simulink model "k1visex"  (Simulink 8.5)
settings: Solver=ode45  StartTime=0.0  StopTime=10.0  RelTol=1e-3
libraries: cdsFilt x6, cdsIPCx x4, cdsEpicsOut x2, cdsAdcx0 x1, dac x1, TYPEC_MASTER x1, cdsParameters x1
settings Model: Creator=controls  LastModifiedBy=controls
settings DataIOCC: SignalLoggingSaveFormat=Dataset
settings OptimizationCC: ExpressionDepthLimit=128
settings DebuggingCC: UnderspecifiedInitializationDetection=Simplified  MergeDetectMultiDrivingBlocksExec=error  FcnCallInpInsideContextMsg=EnableAllAsError  StateNameClashWarn=none
settings GRTTargetCC: CombineOutputUpdateFcns=on  GRTInterface=off

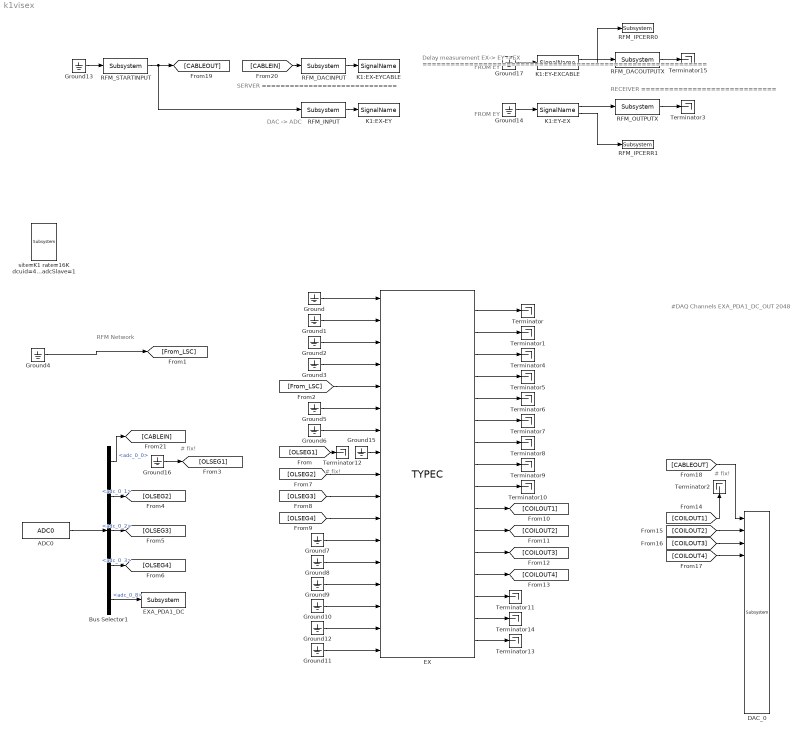
== system k1visex ==
  note: RFM Network
  note: #DAQ Channels
      |
      | EXA_PDA1_DC_OUT 2048
  note: FROM EY
  note: DAC -> ADC
  note: FROM EY
  note: Delay measurement
      | EX-> EY ->EX
      | =============================================================
  note: SERVER
      | =============================
  note: RECEIVER
      | =============================
  note: # fix!
  note: # fix!
  note: # fix!
  ADC0 : cdsAdcx0/ADC0  Tag=cdsAdc  Description=|
      | type-GSC_16AI64SSA
      | card_num=0
      settings: AttributesFormatString=%<Description>\n%<Tag>
  Bus Selector1 : BusSelector  Description=ADC Selector  OutputSignals=adc_0_0,adc_0_1,adc_0_2,adc_0_3,adc_0_8
      settings: AttributesFormatString=%<Description>
  DAC_0 : dac/Subsystem  Description=|
      | type=GSC_16AO16,
      | card_num=0
      settings: AttributesFormatString=%<Description>
  EX : TYPEC_MASTER/TYPEC  Description=TYPEC MASTER
      settings: AttributesFormatString=%<Description>
  EXA_PDA1_DC : cdsFilt/Subsystem  Tag=cdsFilt  Description=|
      | Purpose:                                                                                                                                                                                                                                  
      | Standard CDS IIR filter module.                                                                                                                                                                                                           
      |                                                                                                                                                                                                                                           
      | Operation:                                                                                                                                                                                                                                
      | Consists of 10 second order section IIR filters, plus a ramped gain stage. In FE code, also provides pre-defined test points and excitation channel inputs. The filter coefficients are defined in the LIGO system using the 'foton' tool.
      |                                                                                                                                                                                                                                           
      | Usage:                                                                                                                                                                                                                                    
      | Name the part with the desired filter module name.
      settings: AttributesFormatString=%<Tag>
  Ground{,1..17} (18 alike) : Ground
  K1:EX-EY : cdsIPCx/SignalName  Tag=cdsIPCx_RFM  Description=card=0
      settings: AttributesFormatString=%<Description>\n%<Tag>
  K1:EX-EYCABLE : cdsIPCx/SignalName  Tag=cdsIPCx_RFM  Description=card=0
      settings: AttributesFormatString=%<Description>\n%<Tag>
  K1:EY-EX : cdsIPCx/SignalName  Tag=cdsIPCx_RFM  Description=card=0
      settings: AttributesFormatString=%<Description>\n%<Tag>
  K1:EY-EXCABLE : cdsIPCx/SignalName  Tag=cdsIPCx_RFM  Description=card=0
      settings: AttributesFormatString=%<Description>\n%<Tag>
  RFM_DACINPUT : cdsFilt/Subsystem  Tag=cdsFilt  Description=|
      | Purpose:                                                                                                                                                                                                                                  
      | Standard CDS IIR filter module.                                                                                                                                                                                                           
      |                                                                                                                                                                                                                                           
      | Operation:                                                                                                                                                                                                                                
      | Consists of 10 second order section IIR filters, plus a ramped gain stage. In FE code, also provides pre-defined test points and excitation channel inputs. The filter coefficients are defined in the LIGO system using the 'foton' tool.
      |                                                                                                                                                                                                                                           
      | Usage:                                                                                                                                                                                                                                    
      | Name the part with the desired filter module name.
      settings: AttributesFormatString=%<Tag>
  RFM_DACOUTPUTX : cdsFilt/Subsystem  Tag=cdsFilt  Description=|
      | Purpose:                                                                                                                                                                                                                                  
      | Standard CDS IIR filter module.                                                                                                                                                                                                           
      |                                                                                                                                                                                                                                           
      | Operation:                                                                                                                                                                                                                                
      | Consists of 10 second order section IIR filters, plus a ramped gain stage. In FE code, also provides pre-defined test points and excitation channel inputs. The filter coefficients are defined in the LIGO system using the 'foton' tool.
      |                                                                                                                                                                                                                                           
      | Usage:                                                                                                                                                                                                                                    
      | Name the part with the desired filter module name.
      settings: AttributesFormatString=%<Tag>
  RFM_INPUT : cdsFilt/Subsystem  Tag=cdsFilt  Description=|
      | Purpose:                                                                                                                                                                                                                                  
      | Standard CDS IIR filter module.                                                                                                                                                                                                           
      |                                                                                                                                                                                                                                           
      | Operation:                                                                                                                                                                                                                                
      | Consists of 10 second order section IIR filters, plus a ramped gain stage. In FE code, also provides pre-defined test points and excitation channel inputs. The filter coefficients are defined in the LIGO system using the 'foton' tool.
      |                                                                                                                                                                                                                                           
      | Usage:                                                                                                                                                                                                                                    
      | Name the part with the desired filter module name.
      settings: AttributesFormatString=%<Tag>
  RFM_IPCERR0 : cdsEpicsOut/Subsystem  Tag=cdsEpicsOutput  Description=|
      | Purpose:                                          
      | Output a FE signal to an EPICS channel.           
      |                                                   
      | Operation:                                        
      | Takes input value and passes it to EPICS record.  
      |                                                   
      | Usage:                                            
      | Name the part with the desired EPICS rrecord name.
      settings: AttributesFormatString=%<Tag>
  RFM_IPCERR1 : cdsEpicsOut/Subsystem  Tag=cdsEpicsOutput  Description=|
      | Purpose:                                          
      | Output a FE signal to an EPICS channel.           
      |                                                   
      | Operation:                                        
      | Takes input value and passes it to EPICS record.  
      |                                                   
      | Usage:                                            
      | Name the part with the desired EPICS rrecord name.
      settings: AttributesFormatString=%<Tag>
  RFM_OUTPUTX : cdsFilt/Subsystem  Tag=cdsFilt  Description=|
      | Purpose:                                                                                                                                                                                                                                  
      | Standard CDS IIR filter module.                                                                                                                                                                                                           
      |                                                                                                                                                                                                                                           
      | Operation:                                                                                                                                                                                                                                
      | Consists of 10 second order section IIR filters, plus a ramped gain stage. In FE code, also provides pre-defined test points and excitation channel inputs. The filter coefficients are defined in the LIGO system using the 'foton' tool.
      |                                                                                                                                                                                                                                           
      | Usage:                                                                                                                                                                                                                                    
      | Name the part with the desired filter module name.
      settings: AttributesFormatString=%<Tag>
  RFM_STARTINPUT : cdsFilt/Subsystem  Tag=cdsFilt  Description=|
      | Purpose:                                                                                                                                                                                                                                  
      | Standard CDS IIR filter module.                                                                                                                                                                                                           
      |                                                                                                                                                                                                                                           
      | Operation:                                                                                                                                                                                                                                
      | Consists of 10 second order section IIR filters, plus a ramped gain stage. In FE code, also provides pre-defined test points and excitation channel inputs. The filter coefficients are defined in the LIGO system using the 'foton' tool.
      |                                                                                                                                                                                                                                           
      | Usage:                                                                                                                                                                                                                                    
      | Name the part with the desired filter module name.
      settings: AttributesFormatString=%<Tag>
  Terminator{,1..15} (16 alike) : Terminator
  site=K1 rate=16K dcuid=42 host=k1ex0 specific_cpu=38 adcSlave=1 : cdsParameters/Subsystem  Tag=cdsParameters  Description=|
      | Purpose:                                                                                                                                                                                                                                
      | Provide system parameters to the FE code generator to properly configure the generated EPICS names, rep rate of the FE controller, and the Data Acquisition node ID for proper storage of data from this FE controller.                 
      |                                                                                                                                                                                                                                         
      | Useage:                                                                                                                                                                                                                                 
      | The part NAME field is used to identify the FE parameters. It must be of the form:                                                                                                                                                      
      | site=                                                                                                                                                                                                                                   
      | rate=                                                                                                                                                                                                                                   
      | dcuid=                                                                                                                                                                                                                                  
      |                                                                                                                                                                                                                                         
      | Where:                                                                                                                                                                                                                                  
      | site= argument may be H1, H2, L1, M1, G1, either as a single argument or multiple, for example site=H1,H2. These are the only names allowed. These will become the first two characters of all EPICS and signal names (for example G1:).
      |                                                                                                                                                                                                                                         
      | rate= may be 2K, 16K, 32K, or 64K                                                                                                                                                                                                       
      |                                                                                                                                                                                                                                         
      | dcuid= is site specific ie it must be unique at each site.
      settings: AttributesFormatString=%<Tag>
  wires:
  ADC0/1 -> Bus Selector1/1
  Ground2/1 -> EX/3
  Ground1/1 -> EX/2
  Ground/1 -> EX/1
  Ground3/1 -> EX/4
  Ground8/1 -> EX/13
  Ground7/1 -> EX/12
  Ground9/1 -> EX/14
  Ground10/1 -> EX/15
  Ground5/1 -> EX/6
  Ground12/1 -> EX/16
  Ground11/1 -> EX/17
  EX/1 -> Terminator/1
  EX/2 -> Terminator1/1
  EX/5 -> Terminator6/1
  EX/4 -> Terminator5/1
  EX/6 -> Terminator7/1
  EX/3 -> Terminator4/1
  EX/7 -> Terminator8/1
  EX/9 -> Terminator10/1
  EX/8 -> Terminator9/1
  EX/14 -> Terminator11/1
  EX/15 -> Terminator14/1
  EX/16 -> Terminator13/1
  Ground6/1 -> EX/7
  Bus Selector1/5 -> EXA_PDA1_DC/1  "<adc_0_8>"
  [From_LSC] -> EX/5
  Bus Selector1/1 -> [CABLEIN]  "<adc_0_0>"
  Bus Selector1/2 -> [OLSEG2]  "<adc_0_1>"
  Bus Selector1/3 -> [OLSEG3]  "<adc_0_2>"
  Bus Selector1/4 -> [OLSEG4]  "<adc_0_3>"
  [OLSEG1] -> Terminator12/1
  [OLSEG2] -> EX/9
  [OLSEG3] -> EX/10
  [OLSEG4] -> EX/11
  EX/13 -> [COILOUT4]
  EX/10 -> [COILOUT1]
  EX/11 -> [COILOUT2]
  EX/12 -> [COILOUT3]
  [COILOUT1] -> Terminator2/1
  [COILOUT2] -> DAC_0/2
  [COILOUT3] -> DAC_0/3
  [COILOUT4] -> DAC_0/4
  Ground13/1 -> RFM_STARTINPUT/1
  K1:EY-EX/1 -> RFM_OUTPUTX/1
  K1:EY-EX/2 -> RFM_IPCERR1/1
  Ground14/1 -> K1:EY-EX/1
  RFM_OUTPUTX/1 -> Terminator3/1
  [CABLEOUT] -> DAC_0/1
  Ground15/1 -> EX/8
  Ground16/1 -> [OLSEG1]
  [CABLEIN] -> RFM_DACINPUT/1
  K1:EY-EXCABLE/1 -> RFM_DACOUTPUTX/1
  K1:EY-EXCABLE/2 -> RFM_IPCERR0/1
  Ground17/1 -> K1:EY-EXCABLE/1
  RFM_DACOUTPUTX/1 -> Terminator15/1
  RFM_DACINPUT/1 -> K1:EX-EYCABLE/1
  RFM_INPUT/1 -> K1:EX-EY/1
  RFM_STARTINPUT/1 -> RFM_INPUT/1, [CABLEOUT]
  Ground4/1 -> [From_LSC]
